simulink model "untitled1"  (R2020b)
settings: Solver=VariableStepAuto  StartTime=0.0  StopTime=10.0  RelTol=1e-3
values from neighbouring files (symbols this model uses):
  waypoints = [0  0; 4  2; 3  7; -3  6]    [matlab.mat]
undefined symbols (not defined in the file or in its folder): duration, effort, index, joint_name, left_wheel_hinge, model_name, pioneer2dx, right_wheel_hinge
libraries: robotgazebolib x11, robotalgslib x1, robotcorelib x1
settings Model: Creator=tfpeng  LastModifiedBy=tfpeng

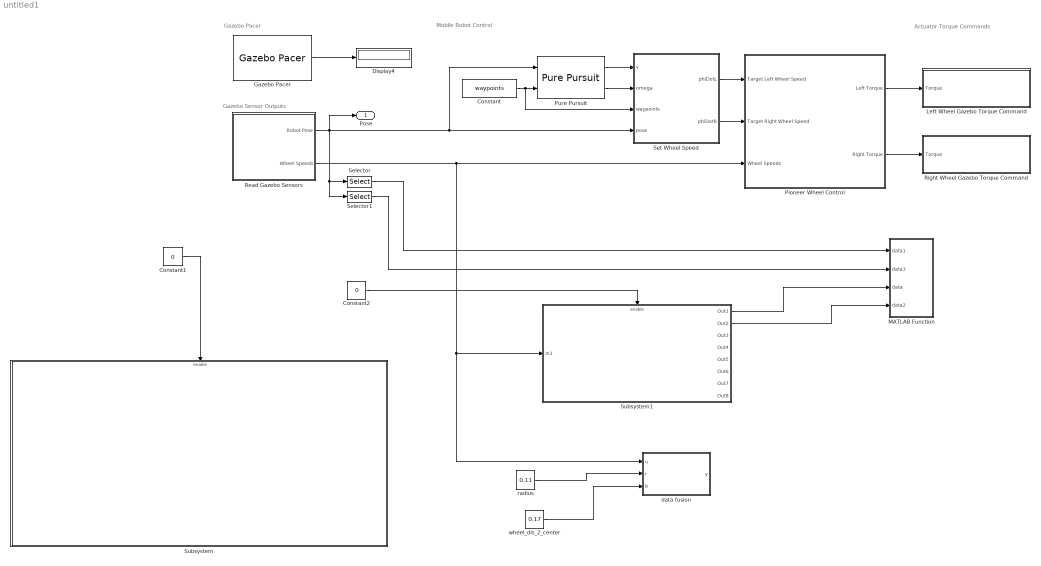
== system untitled1 ==
  note: Gazebo Pacer
  note: Actuator Torque Commands
  note: Mobile Robot Control
  note: Gazebo Sensor Outputs
  Constant : Constant  Value=waypoints
  Constant1 : Constant  Value=0
  Constant2 : Constant  Value=0
  Display4 : Display
  Gazebo Pacer : robotgazebolib/Gazebo Pacer  ResetBehavior=Reset Gazebo simulation time and scene  SampleTime=0.01
      settings: SourceProductName=Robotics System Toolbox
  Left Wheel Gazebo Torque Command : Subsystem
  MATLAB Function : MATLAB Function  TreatAsAtomicUnit=on
  Pioneer Wheel Control : Subsystem
  Pure Pursuit : robotalgslib/Pure Pursuit  DesiredLinearVelocity=1  MaxAngularVelocity=1.0  LookaheadDistance=1.0  TargetDirPort=off  SimulateUsing=Code generation
  Read Gazebo Sensors : Subsystem
  Right Wheel Gazebo Torque Command : Subsystem
  Selector : Selector  InputPortWidth=3  IndexOptions=Index vector (dialog)  Indices=[1]  OutputSizes=1
  Selector1 : Selector  InputPortWidth=3  IndexOptions=Index vector (dialog)  Indices=[2]  OutputSizes=1
  Set Wheel Speed : MATLAB Function  TreatAsAtomicUnit=on
  Subsystem : Subsystem
  Subsystem1 : Subsystem
  data fusion : Subsystem  TreatAsAtomicUnit=on
  radius : Constant  Value=0.11
  wheel_dis_2_center : Constant  Value=0.17
  Pose : Outport
  wires:
  Pure Pursuit/2 -> Set Wheel Speed/2(omega)
  Selector/1 -> MATLAB Function/1(data1)
  Constant/1 -> Set Wheel Speed/3(waypoints), Pure Pursuit/2
  Gazebo Pacer/1 -> Display4/1
  Selector1/1 -> MATLAB Function/2(data3)
  Read Gazebo Sensors/2(Wheel Speeds) -> Subsystem1/1(In1), data fusion/1(u), Pioneer Wheel Control/3(Wheel Speeds)
  Pioneer Wheel Control/2(Right Torque) -> Right Wheel Gazebo Torque Command/1(Torque)
  Pure Pursuit/1 -> Set Wheel Speed/1(v)
  Read Gazebo Sensors/1(Robot Pose) -> Pose/1, Selector/1, Selector1/1, Pure Pursuit/1, Set Wheel Speed/4(pose)
  Set Wheel Speed/2(phiDotR) -> Pioneer Wheel Control/2(Target Right Wheel Speed)
  Set Wheel Speed/1(phiDotL) -> Pioneer Wheel Control/1(Target Left Wheel Speed)
  Pioneer Wheel Control/1(Left Torque) -> Left Wheel Gazebo Torque Command/1(Torque)
  Constant1/1 -> Subsystem/Enable
  Subsystem1/1(Out1) -> MATLAB Function/3(data)
  Subsystem1/2(Out2) -> MATLAB Function/4(data2)
  Constant2/1 -> Subsystem1/Enable
  radius/1 -> data fusion/2(r)
  wheel_dis_2_center/1 -> data fusion/3(b)

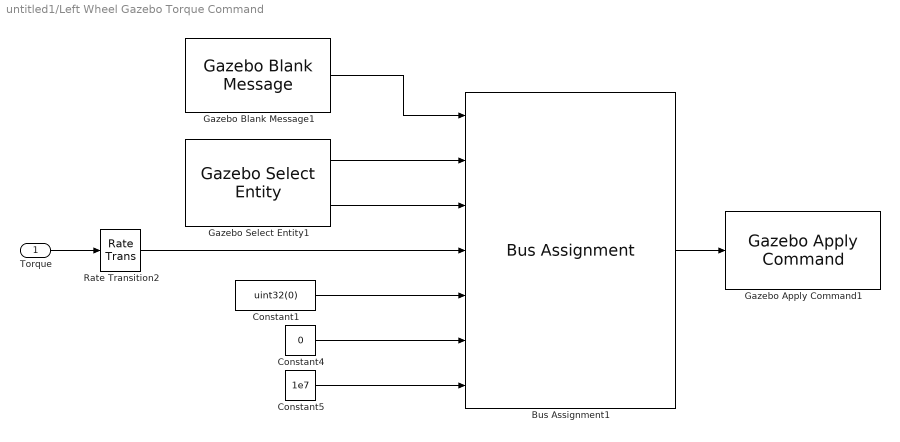
== system untitled1/Left Wheel Gazebo Torque Command ==
  Torque : Inport
  Bus Assignment1 : BusAssignment  AssignedSignals=model_name,joint_name,effort,index,duration.seconds,duration.nano_seconds
  Constant1 : Constant  Value=uint32(0)
  Constant4 : Constant  Value=0
  Constant5 : Constant  Value=1e7
  Gazebo Apply Command1 : robotgazebolib/Gazebo Apply Command  cmdType=ApplyJointTorque  sampleTime=0.01
      settings: SourceProductName=Robotics System Toolbox
  Gazebo Blank Message1 : robotgazebolib/Gazebo Blank Message  msgType=ApplyJointTorque  sampleTime=0.01  busName='Gazebo_SL_Bus_gazebo_msgs_ApplyJointTorque'
      settings: SourceProductName=Robotics System Toolbox
  Gazebo Select Entity1 : robotgazebolib/Gazebo Select Entity  modelElemName=pioneer2dx/left_wheel_hinge  outputArraySize=128  OutputLabel=Joint  SelectType=Joint
      settings: SourceProductName=Robotics System Toolbox
  Rate Transition2 : RateTransition
  wires:
  Bus Assignment1/1 -> Gazebo Apply Command1/1
  Constant5/1 -> Bus Assignment1/7
  Gazebo Blank Message1/1 -> Bus Assignment1/1
  Gazebo Select Entity1/2 -> Bus Assignment1/3
  Gazebo Select Entity1/1 -> Bus Assignment1/2
  Torque/1 -> Rate Transition2/1
  Constant4/1 -> Bus Assignment1/6
  Rate Transition2/1 -> Bus Assignment1/4
  Constant1/1 -> Bus Assignment1/5

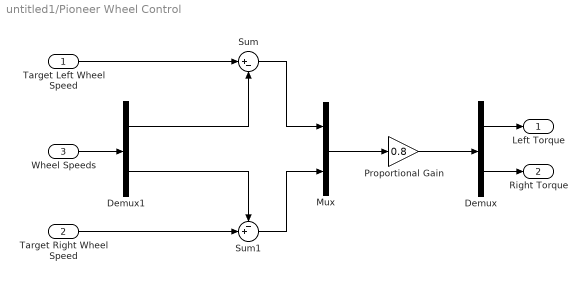
== system untitled1/Pioneer Wheel Control ==
  Target Left Wheel Speed : Inport
  Target Right Wheel Speed : Inport  Port=2
  Wheel Speeds : Inport  Port=3
  Demux : Demux  Outputs=2
  Demux1 : Demux  Outputs=2
  Mux : Mux  Inputs=2
  Proportional Gain : Gain  Gain=0.8
  Sum : Sum  Inputs=|+-
  Sum1 : Sum  Inputs=-+|
  Left Torque : Outport
  Right Torque : Outport  Port=2
  wires:
  Sum1/1 -> Mux/2
  Target Left Wheel Speed/1 -> Sum/1
  Sum/1 -> Mux/1
  Mux/1 -> Proportional Gain/1
  Proportional Gain/1 -> Demux/1
  Demux/1 -> Left Torque/1
  Demux/2 -> Right Torque/1
  Wheel Speeds/1 -> Demux1/1
  Demux1/1 -> Sum/2
  Target Right Wheel Speed/1 -> Sum1/2
  Demux1/2 -> Sum1/1

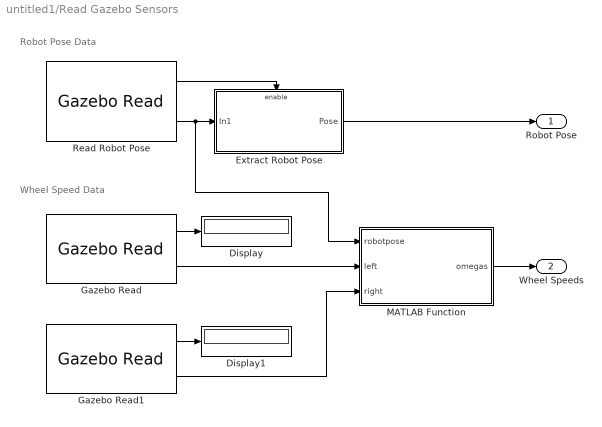
== system untitled1/Read Gazebo Sensors ==
  note: Robot Pose Data
  note: Wheel Speed Data
  Display : Display
  Display1 : Display
  Extract Robot Pose : Subsystem
  Gazebo Read : robotgazebolib/Gazebo Read  topicSource=From Gazebo  topic=/gazebo/ground_truth/world_pose/pioneer2dx/left_wheel  messageType=gazebo_msgs/Pose  sampleTime=0.01
      settings: SourceProductName=Robotics System Toolbox
  Gazebo Read1 : robotgazebolib/Gazebo Read  topicSource=From Gazebo  topic=/gazebo/ground_truth/world_pose/pioneer2dx/right_wheel  messageType=gazebo_msgs/Pose  sampleTime=0.01
      settings: SourceProductName=Robotics System Toolbox
  MATLAB Function : MATLAB Function  TreatAsAtomicUnit=on
  Read Robot Pose : robotgazebolib/Gazebo Read  topicSource=From Gazebo  topic=/gazebo/ground_truth/world_pose/pioneer2dx/chassis  messageType=gazebo_msgs/Pose  sampleTime=0.01
      settings: SourceProductName=Robotics System Toolbox
  Robot Pose : Outport
  Wheel Speeds : Outport  Port=2
  wires:
  Read Robot Pose/2 -> MATLAB Function/1(robotpose), Extract Robot Pose/1(In1)
  Extract Robot Pose/1(Pose) -> Robot Pose/1
  Read Robot Pose/1 -> Extract Robot Pose/Enable
  Gazebo Read/1 -> Display/1
  Gazebo Read1/1 -> Display1/1
  MATLAB Function/1(omegas) -> Wheel Speeds/1
  Gazebo Read/2 -> MATLAB Function/2(left)
  Gazebo Read1/2 -> MATLAB Function/3(right)

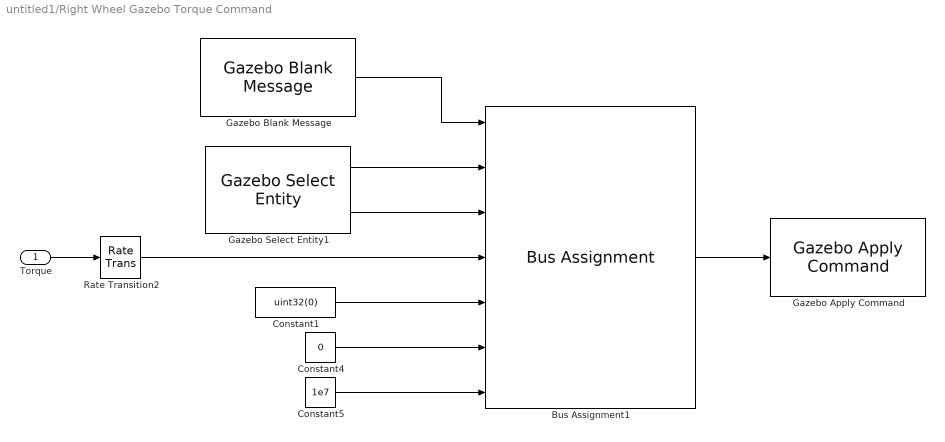
== system untitled1/Right Wheel Gazebo Torque Command ==
  Torque : Inport
  Bus Assignment1 : BusAssignment  AssignedSignals=model_name,joint_name,effort,index,duration.seconds,duration.nano_seconds
  Constant1 : Constant  Value=uint32(0)
  Constant4 : Constant  Value=0
  Constant5 : Constant  Value=1e7
  Gazebo Apply Command : robotgazebolib/Gazebo Apply Command  cmdType=ApplyJointTorque  sampleTime=0.01
      settings: SourceProductName=Robotics System Toolbox
  Gazebo Blank Message : robotgazebolib/Gazebo Blank Message  msgType=ApplyJointTorque  sampleTime=0.01  busName='Gazebo_SL_Bus_gazebo_msgs_ApplyJointTorque'
      settings: SourceProductName=Robotics System Toolbox
  Gazebo Select Entity1 : robotgazebolib/Gazebo Select Entity  modelElemName=pioneer2dx/right_wheel_hinge  outputArraySize=128  OutputLabel=Joint  SelectType=Joint
      settings: SourceProductName=Robotics System Toolbox
  Rate Transition2 : RateTransition
  wires:
  Constant1/1 -> Bus Assignment1/5
  Rate Transition2/1 -> Bus Assignment1/4
  Constant4/1 -> Bus Assignment1/6
  Torque/1 -> Rate Transition2/1
  Gazebo Select Entity1/1 -> Bus Assignment1/2
  Gazebo Select Entity1/2 -> Bus Assignment1/3
  Gazebo Blank Message/1 -> Bus Assignment1/1
  Constant5/1 -> Bus Assignment1/7
  Bus Assignment1/1 -> Gazebo Apply Command/1

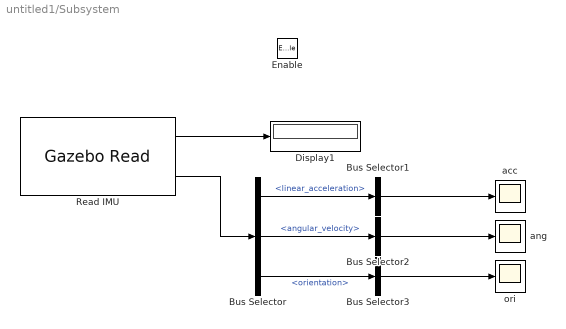
== system untitled1/Subsystem ==
  Enable : EnablePort
  Bus Selector : BusSelector  OutputSignals=linear_acceleration,angular_velocity,orientation
  Bus Selector1 : BusSelector  OutputSignals=x,y,z  OutputAsBus=on
  Bus Selector2 : BusSelector  OutputSignals=x,y,z  OutputAsBus=on
  Bus Selector3 : BusSelector  OutputSignals=w,x,y,z  OutputAsBus=on
  Display1 : Display
  Read IMU : robotgazebolib/Gazebo Read  topicSource=From Gazebo  topic=/gazebo/default/pioneer2dx/chassis/imu/imu  messageType=gazebo_msgs/IMU  sampleTime=0.01
      settings: SourceProductName=Robotics System Toolbox
  acc : Scope
  ang : Scope
  ori : Scope
  wires:
  Bus Selector2/1 -> ang/1
  Read IMU/1 -> Display1/1
  Read IMU/2 -> Bus Selector/1
  Bus Selector3/1 -> ori/1
  Bus Selector/3 -> Bus Selector3/1  "<orientation>"
  Bus Selector/1 -> Bus Selector1/1  "<linear_acceleration>"
  Bus Selector1/1 -> acc/1
  Bus Selector/2 -> Bus Selector2/1  "<angular_velocity>"

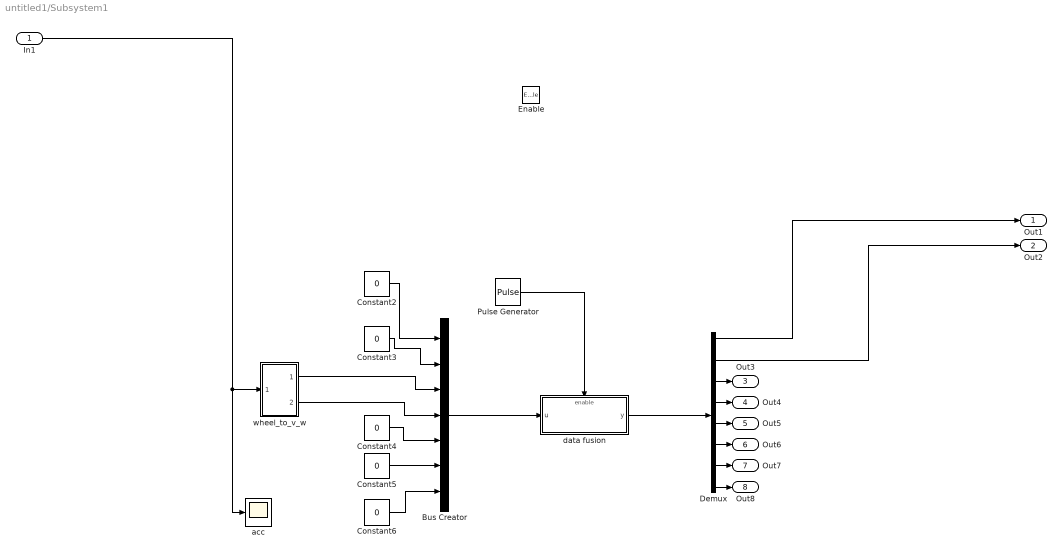
== system untitled1/Subsystem1 ==
  In1 : Inport
  Enable : EnablePort
  Bus Creator : BusCreator  Inputs=7
  Constant{2..6} (5 alike) : Constant  Value=0
  Demux : Demux  Outputs=8
  Pulse Generator : DiscretePulseGenerator  PulseType=Time based  Period=0.01  PulseWidth=50
  acc : Scope
  data fusion : Subsystem  TreatAsAtomicUnit=on
  wheel_to_v_w : Subsystem
  Out1 : Outport
  Out2 : Outport  Port=2
  Out3 : Outport  Port=3
  Out4 : Outport  Port=4
  Out5 : Outport  Port=5
  Out6 : Outport  Port=6
  Out7 : Outport  Port=7
  Out8 : Outport  Port=8
  wires:
  wheel_to_v_w/1(Out1) -> Bus Creator/3
  Demux/7 -> Out7/1
  Demux/8 -> Out8/1
  wheel_to_v_w/2(Out2) -> Bus Creator/4
  Pulse Generator/1 -> data fusion/Enable
  Constant3/1 -> Bus Creator/2
  Demux/2 -> Out2/1
  Constant4/1 -> Bus Creator/5
  Demux/3 -> Out3/1
  Constant6/1 -> Bus Creator/7
  In1/1 -> acc/1, wheel_to_v_w/1(In1)
  Constant5/1 -> Bus Creator/6
  Constant2/1 -> Bus Creator/1
  data fusion/1(y) -> Demux/1
  Demux/4 -> Out4/1
  Demux/1 -> Out1/1
  Demux/5 -> Out5/1
  Bus Creator/1 -> data fusion/1(u)
  Demux/6 -> Out6/1

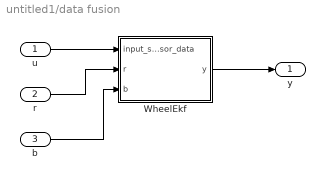
== system untitled1/data fusion ==
  u : Inport
  r : Inport  Port=2
  b : Inport  Port=3
  WheelEkf : MATLAB Function  TreatAsAtomicUnit=on
  y : Outport
  wires:
  u/1 -> WheelEkf/1(input_sensor_data)
  WheelEkf/1(y) -> y/1
  r/1 -> WheelEkf/2(r)
  b/1 -> WheelEkf/3(b)

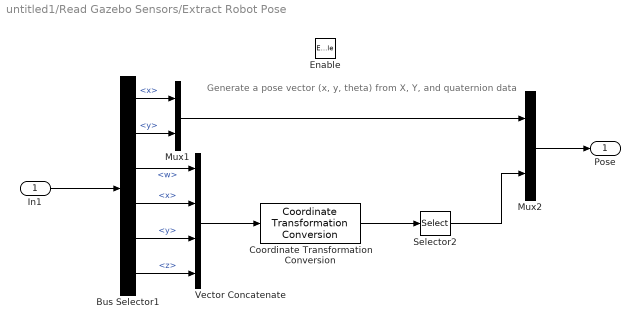
== system untitled1/Read Gazebo Sensors/Extract Robot Pose ==
  note: Generate a pose vector (x, y, theta) from X, Y, and quaternion data
  In1 : Inport
  Enable : EnablePort
  Bus Selector1 : BusSelector  OutputSignals=position.x,position.y,orientation.w,orientation.x,orientation.y,orientation.z
  Coordinate Transformation Conversion : robotcorelib/Coordinate Transformation Conversion  InputRepresentation=Quaternion  InputEulerSequence=ZYX  ShowTrVecInputPort=on  OutputRepresentation=Euler Angles  OutputEulerSequence=ZYX  ShowTrVecOutputPort=on  SimulateUsing=Interpreted execution
  Mux1 : Mux  Inputs=2
  Mux2 : Mux  Inputs=2
  Selector2 : Selector  InputPortWidth=3  IndexOptions=Index vector (dialog)  Indices=1  OutputSizes=1
  Vector Concatenate : Concatenate  NumInputs=4
  Pose : Outport  VectorParamsAs1DForOutWhenUnconnected=off
  wires:
  Vector Concatenate/1 -> Coordinate Transformation Conversion/1
  Coordinate Transformation Conversion/1 -> Selector2/1
  Mux1/1 -> Mux2/1
  Selector2/1 -> Mux2/2
  Mux2/1 -> Pose/1
  Bus Selector1/6 -> Vector Concatenate/4  "<z>"
  Bus Selector1/1 -> Mux1/1  "<x>"
  Bus Selector1/4 -> Vector Concatenate/2  "<x>"
  Bus Selector1/2 -> Mux1/2  "<y>"
  Bus Selector1/3 -> Vector Concatenate/1  "<w>"
  Bus Selector1/5 -> Vector Concatenate/3  "<y>"
  In1/1 -> Bus Selector1/1

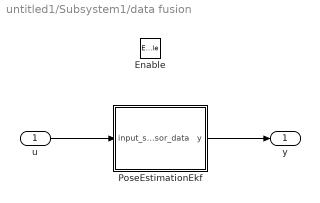
== system untitled1/Subsystem1/data fusion ==
  u : Inport
  Enable : EnablePort
  PoseEstimationEkf : MATLAB Function  TreatAsAtomicUnit=on
  y : Outport
  wires:
  u/1 -> PoseEstimationEkf/1(input_sensor_data)
  PoseEstimationEkf/1(y) -> y/1

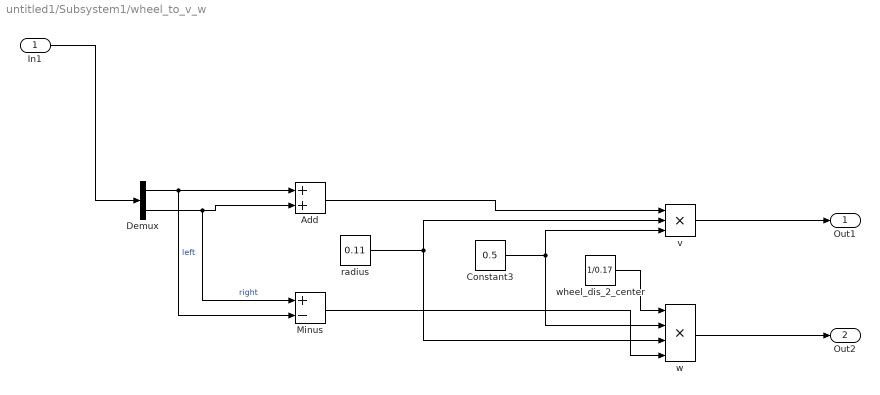
== system untitled1/Subsystem1/wheel_to_v_w ==
  In1 : Inport
  Add : Sum
  Constant3 : Constant  Value=0.5
  Demux : Demux  Outputs=2
  Minus : Sum  Inputs=+-
  radius : Constant  Value=0.11
  v : Product  Inputs=3
  w : Product  Inputs=4
  wheel_dis_2_center : Constant  Value=1/0.17
  Out1 : Outport
  Out2 : Outport  Port=2
  wires:
  Minus/1 -> w/4
  w/1 -> Out2/1
  In1/1 -> Demux/1
  Add/1 -> v/1
  wheel_dis_2_center/1 -> w/1
  v/1 -> Out1/1
  radius/1 -> w/3, v/2
  Demux/2 -> Minus/1, Add/2  "right"
  Demux/1 -> Minus/2, Add/1  "left"
  Constant3/1 -> w/2, v/3

== matlab function untitled1/Read Gazebo Sensors/MATLAB Function ==
  data: robotpose input; omegas output; left input; right input
function omegas = computeWheelVelocities(robotpose, left, right)
%computeWheelVelocities computes wheel velocity based on rate of change of
%the yaw angle of the wheel relative to its original mount on the robot
%body

persistent initAngles
if isempty(initAngles)
    initAngles = zeros(2,1);
end
sampleTime = 0.01;

% compute rotation between wheel original mount on the robot body and world
% frame
robotRtom = quat2rotm([robotpose.orientation.w, robotpose.orientation.x, robotpose.orientation.y, robotpose.orientation.z]);
originalWheelMount = robotRtom*eul2rotm([pi/2 pi/2 0]);

% get rotation between wheel and the world frame
leftRtom = quat2rotm([left.orientation.w, left.orientation.x, left.orientation.y, left.orientation.z]);
rightRtom = quat2rotm([right.orientation.w, right.orientation.x, right.orientation.y, right.orientation.z]);

% compute relative rotation between wheel and its original mount
leftRotation = rotm2eul(originalWheelMount'*leftRtom);
rightRotation = rotm2eul(originalWheelMount'*rightRtom);

% compute angluar velocity using the angle difference between the current
% angle pose and the the angle pose in last time step
angles = [leftRotation(1); rightRotation(1)];
omegas = angdiff(initAngles, angles)/sampleTime;
initAngles = angles;

== matlab function untitled1/Set Wheel Speed ==
  data: v input; omega input; waypoints input; pose input; phiDotL output; phiDotR output
function [phiDotL, phiDotR] = wheelSpeed(v, omega, waypoints, pose)

% Path constants
stopThreshold = 0.1;
slowThreshold = 0.3;

% Robot constants
trackWidth = 0.381;
wheelRadius = 0.195/2;

% Slow the robot down when it's near the threshold
distanceToEndpoint = norm(waypoints(end, :) - pose(1:2)');
if (distanceToEndpoint < slowThreshold)
    v = distanceToEndpoint/slowThreshold*v;
    
    % Stop the robot if it's inside the target threshold
    if distanceToEndpoint < stopThreshold
        v = 0;
    end
end

% Convert velocity and heading angular velocity to wheel speeds
phiDotL = (v - trackWidth/2*omega)/wheelRadius;
phiDotR = (v + trackWidth/2*omega)/wheelRadius;

end

== matlab function untitled1/Subsystem1/data fusion/PoseEstimationEkf ==
  data: input_sensor_data input; y output
function y = PoseEstimationEkf(input_sensor_data)
persistent state_variable_current state_variable_last P Q;
if isempty(state_variable_current)
        state_variable_current=zeros(8,1);
        state_variable_last=zeros(8,1);
        Q=diag([0.1, 0.1, 0.1,0.1, 0.1, 0.1, 0.1, 0.1]);
        P=Q;
end
persistent time_ms;
if isempty(time_ms)
    time_ms=tic;
    y=state_variable_current;
    return;
end
%%    predict
dt=0.01;
A=[[1, 0, 0, dt, 0, 0, 0.5*dt^2, 0]
  [0, 1, 0, 0, dt, 0, 0, 0.5*dt^2]
  [0, 0, 1, 0, 0, dt, 0, 0]
  [0, 0, 0, 1, 0, 0, dt, 0]
  [0, 0, 0, 0, 1, 0, 0, dt]
  [0, 0, 0, 0, 0, 1, 0, 0]
  [0, 0, 0, 0, 0, 0, 1, 0]
  [0, 0, 0, 0, 0, 0, 0, 1]];
state_variable_current=A*state_variable_current;
P=A*P*A'+Q;

%%    update
theta = state_variable_current(3);
vx = state_variable_current(4);
vy = state_variable_current(5);
v = sqrt(vx^2+vy^2);
w = state_variable_current(6);
H=[[0, 0, 0, 0, 0, 0, 0, 0]
  [0, 0, 0, 0, 0, 0, 0, 0]
  [0, 0, 0, cos(theta), sin(theta), 0, 0, 0]
  [0, 0, 0, 0, 0, 1, 0, 0]
  [0, 0, 0, 0, 0, 0, 0, 0]
  [0, 0, 0, 0, 0, 0, 0, 0]
  [0, 0, 0, 0, 0, 0, 0, 0]];
Z=[0, 0, v, w, 0, 0, 0]';
R = diag([0.01, 0.01, 0.001, 0.001, 0.01, 0.01, 0.01]);
error=input_sensor_data-Z;

temp_p=H*P*H'+R;
kalman_gain=(P*H')/(temp_p);
correct_value=kalman_gain*error;
state_variable_current=state_variable_current+correct_value;
P=P-kalman_gain*H*P;

time_ms=tic;
y = state_variable_current;

== matlab function untitled1/MATLAB Function ==
  data: data1 input; data3 input; data input; data2 input
function fcn(data1, data3, data, data2)
persistent data1arr data2arr

if isempty(data1arr)
    data1arr=[0,0];
end

if isempty(data2arr)
    data2arr=[0,0];
end

data1arr=[data1arr;[data1 data3]];
data2arr=[data2arr;[data data2]];
plot(data1arr(:,1),data1arr(:,2));
hold on;
plot(data2arr(:,1),data2arr(:,2));
hold on;

== matlab function untitled1/data fusion/WheelEkf ==
  data: input_sensor_data input; y output; r input; b input
function y = WheelEkf(input_sensor_data,r,b)
persistent state_variable_current state_variable_last P Q;
if isempty(state_variable_current)
        state_variable_current=zeros(5,1);%[x,y,vx,vy,theta]
        state_variable_last=zeros(5,1);
        Q=diag([0.1, 0.1, 0.1, 0.1, 0.1]);
        P=Q;
end
persistent time_ms;
if isempty(time_ms)
    time_ms=tic;
    y=state_variable_current;
    return;
end
%%    predict
dt=0.01;
A=[[1, 0, dt, 0, 0]
  [0, 1, 0, dt, 0 ]
  [0, 0, 1, 0, 0]
  [0, 0, 0, 1, 0]
  [0, 0, 0, 0, 1]
  ];
state_variable_current=A*state_variable_current;
P=A*P*A'+Q;

%%    update
theta = state_variable_current(5);
d=sqrt(state_variable_current(1)^2+state_variable_current(1)^2);
H=[[0,0,cos(theta),sin(theta),0]
    [0,0,cos(theta),sin(theta),0]];
Z=[d/r/dt,d/r/dt]';
R = diag([0.01, 0.01, 0.01, 0.01, 0.01]);
error=input_sensor_data-Z;

temp_p=H*P*H'+R;
kalman_gain=(P*H')/(temp_p);
correct_value=kalman_gain*error;
state_variable_current=state_variable_current+correct_value;
P=P-kalman_gain*H*P;

time_ms=tic;
y = state_variable_current;
